simulink model "G431_ADC"  (R2018b)
settings: Solver=FixedStepDiscrete  StartTime=0.0  StopTime=10.0  FixedStep=0.010  RelTol=1e-3  EnableMultiTasking=on
libraries: ADC_Lib x2, USART_Lib x2, STM32_Config_Lib x1
settings Model: Creator=reynaudp  LastModifiedBy=fenard1
settings DataIOCC: LimitDataPoints=on  SaveFormat=Array
settings OptimizationCC: DefaultParameterBehavior=Inlined  DefaultUnderspecifiedDataType=single  LifeSpan=1
settings DebuggingCC: UnderspecifiedInitializationDetection=Classic  MergeDetectMultiDrivingBlocksExec=none  SolverPrmCheckMsg=warning  UniqueDataStoreMsg=error  AllowSymbolicDim=off  StrictBusMsg=ErrorOnBusTreatedAsVector  SFUnexpectedBacktrackingDiag=warning  SFNoUnconditionalDefaultTransitionDiag=warning  SFUndirectedBroadcastEventsDiag=error  SFExecutionAtInitializationDiag=none
settings HardwareCC: ProdBitPerPointer=32  ProdBitPerSizeT=32  ProdBitPerPtrDiffT=32  ProdLargestAtomicInteger=Integer  ProdWordSize=32  ProdHWDeviceType=STMicroelectronics->STM32 32-bit Cortex-M  TargetBitPerPointer=64  TargetBitPerSizeT=64  TargetBitPerPtrDiffT=64  TargetLongLongMode=on  TargetIntDivRoundTo=Zero  TargetEndianess=LittleEndian  TargetWordSize=64  TargetHWDeviceType=MATLAB Host  ProdEqTarget=off
settings ModelReferenceCC: PropagateSignalLabelsOutOfModel=off
settings SFSimCC: SimUseLocalCustomCode=off  CompileTimeRecursionLimit=0  EnableRuntimeRecursion=off  MATLABDynamicMemAlloc=off
settings RTWCC: SystemTargetFile=stm32.tlc  TemplateMakefile=stm32.tmf  Description=stm32 (Embedded Target)  GenerateReport=on  RTWUseLocalCustomCode=off  IncludeHyperlinkInReport=on
settings CodeAppCC: IgnoreCustomStorageClasses=off  CustomSymbolStrType=$N$R$M  SimulinkBlockComments=off
settings STFCustomTargetCC: ParMdlRefBuildCompliant=on  IncludeMdlTerminateFcn=off  CombineOutputUpdateFcns=on  ERTCustomFileBanners=on  SupportComplex=off  SupportContinuousTime=off  SupportNonInlinedSFcns=off  RemoveResetFunc=on  ParenthesesLevel=Maximum  CastingMode=Standards  MATLABClassNameForMDSCustomization=Simulink.SoftwareTarget.ERTCustomization  SystemTargetFile=stm32.tlc
settings ERTTargetCC: MultiwordLength=2048  CompOptLevelCompliant=off  ConcurrentExecutionCompliant=off  IncludeMdlTerminateFcn=off  SupportComplex=off  ParenthesesLevel=Maximum  CastingMode=Standards  ModelStepFunctionPrototypeControlCompliant=off  CPPClassGenCompliant=off  UseToolchainInfoCompliant=off  ERTSrcFileBannerTemplate=sourceFileTemplate.cgt  ERTHdrFileBannerTemplate=sourceFileTemplate.cgt  ERTDataSrcFileTemplate=sourceFileTemplate.cgt  ERTDataHdrFileTemplate=sourceFileTemplate.cgt  ERTCustomFileTemplate=customRoutineProcess.tlc  ConvertIfToSwitch=off  SuppressUnreachableDefaultCases=off
settings ConfigComp: CovMetricSettings=dw  CovHtmlReporting=on  CovSaveCumulativeToWorkspaceVar=on  CovSaveSingleToWorkspaceVar=on  CovExternalEMLEnable=off  CovSFcnEnable=off

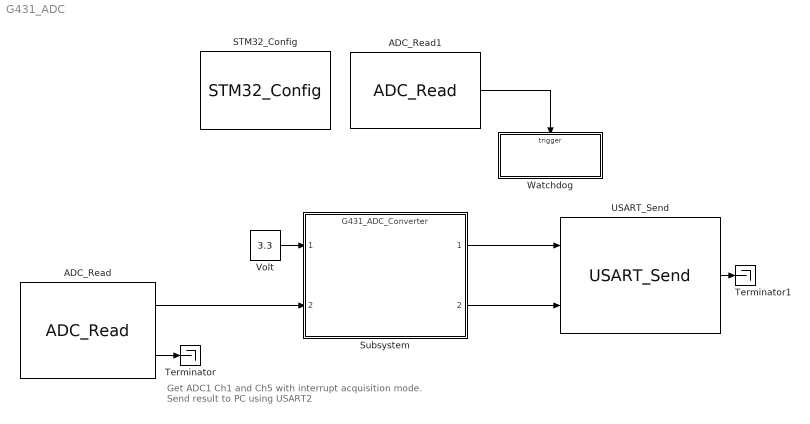
== system G431_ADC ==
  note: Get ADC1 Ch1 and Ch5 with interrupt acquisition mode.
      | Send result to PC using USART2
  ADC_Read : ADC_Lib/ADC_Read  ADC_Name=ADC1  ADC_Ch0=off  ADC_Ch1=on  ADC_Ch2=off  ADC_Ch3=off  ADC_Ch4=off  ADC_Ch5=on  ADC_Ch6=off  ADC_Ch7=off  ADC_Ch8=off  ADC_Ch9=off  ADC_Ch10=off  ADC_Ch11=off  ADC_Ch12=off  ADC_Ch13=off  ADC_Ch14=off  ADC_Ch15=off  ADC_Ch16=off  ADC_Ch17=off  ADC_Ch18=off  RgRk1=on  RgRk2=on  RgRk3=off  RgRk4=off  RgRk1_Ch=Ch1_r1  RgRk2_Ch=Ch5_r2  RgRk3_Ch=off  RgRk4_Ch=off  RgRk5=off  RgRk6=off  RgRk7=off  RgRk8=off  RgRk5_Ch=off  RgRk6_Ch=off  RgRk7_Ch=off  RgRk8_Ch=off  RgRk9=off  RgRk10=off  RgRk11=off  RgRk12=off  RgRk9_Ch=off  RgRk10_Ch=off  RgRk11_Ch=off  RgRk12_Ch=off  RgRk13=off  RgRk14=off  RgRk15=off  RgRk16=off  RgRk13_Ch=off  RgRk14_Ch=off  RgRk15_Ch=off  RgRk16_Ch=off  InjRk1=off  InjRk2=off  InjRk3=off  InjRk4=off  InjRk1_Ch=off  InjRk2_Ch=off  InjRk3_Ch=off  InjRk4_Ch=off  ADC_Trig=Not used  ADC_TrigEdge=Not used  DmaReq=off  DMA_Buffer=0  ItReq=on  AWD_Mode=SINGLE_REG  AWD_Ch=1  AWD_HThres=2000  AWD_LThres=500  AWD_En_Int=on  AWD2_HThres=0  AWD2_LThres=0  AWD2_En_Int=off  AWD3_HThres=0  AWD3_LThres=0  AWD3_En_Int=off  EOC_SEQ=off  EOC_IT=off  JEOC_IT=off  AWD_IT=off  OVR_IT=off  CpltTrans=off  HalfTrans=off  ADC_RegNb=2  ADC_RegCh0=off  ADC_RegCh1=on  ADC_RegCh2=off  ADC_RegCh3=off  ADC_RegCh4=off  ADC_RegCh5=on  ADC_RegCh6=off  ADC_RegCh7=off  ADC_RegCh8=off  ADC_RegCh9=off  ADC_RegCh10=off  ADC_RegCh11=off  ADC_RegCh12=off  ADC_RegCh13=off  ADC_RegCh14=off  ADC_RegCh15=off  ADC_RegCh16=off  ADC_RegCh17=off  ADC_RegCh18=off  ADC_InjNb=0  ADC_InjCh0=off  ADC_InjCh1=off  ADC_InjCh2=off  ADC_InjCh3=off  ADC_InjCh4=off  ADC_InjCh5=off  ADC_InjCh6=off  ADC_InjCh7=off  ADC_InjCh8=off  ADC_InjCh9=off  ADC_InjCh10=off  ADC_InjCh11=off  ADC_InjCh12=off  ADC_InjCh13=off  ADC_InjCh14=off  ADC_InjCh15=off  ADC_InjCh16=off  ADC_InjCh17=off  ADC_InjCh18=off  NbADC=1  CurrentADC=ADC1
      settings: SourceProductName=Target Support Package - STM32 Adapter
  ADC_Read1 : ADC_Lib/ADC_Read  ADC_Name=ADC1  ADC_Ch0=off  ADC_Ch1=off  ADC_Ch2=off  ADC_Ch3=off  ADC_Ch4=off  ADC_Ch5=off  ADC_Ch6=off  ADC_Ch7=off  ADC_Ch8=off  ADC_Ch9=off  ADC_Ch10=off  ADC_Ch11=off  ADC_Ch12=off  ADC_Ch13=off  ADC_Ch14=off  ADC_Ch15=off  ADC_Ch16=off  ADC_Ch17=off  ADC_Ch18=off  RgRk1=off  RgRk2=off  RgRk3=off  RgRk4=off  RgRk1_Ch=Ch1_r1  RgRk2_Ch=Ch5_r2  RgRk3_Ch=off  RgRk4_Ch=off  RgRk5=off  RgRk6=off  RgRk7=off  RgRk8=off  RgRk5_Ch=off  RgRk6_Ch=off  RgRk7_Ch=off  RgRk8_Ch=off  RgRk9=off  RgRk10=off  RgRk11=off  RgRk12=off  RgRk9_Ch=off  RgRk10_Ch=off  RgRk11_Ch=off  RgRk12_Ch=off  RgRk13=off  RgRk14=off  RgRk15=off  RgRk16=off  RgRk13_Ch=off  RgRk14_Ch=off  RgRk15_Ch=off  RgRk16_Ch=off  InjRk1=off  InjRk2=off  InjRk3=off  InjRk4=off  InjRk1_Ch=off  InjRk2_Ch=off  InjRk3_Ch=off  InjRk4_Ch=off  ADC_Trig=Not used  ADC_TrigEdge=Not used  DmaReq=off  DMA_Buffer=0  ItReq=on  AWD_Mode=SINGLE_REG  AWD_Ch=1  AWD_HThres=2000  AWD_LThres=500  AWD_En_Int=on  AWD2_HThres=0  AWD2_LThres=0  AWD2_En_Int=off  AWD3_HThres=0  AWD3_LThres=0  AWD3_En_Int=off  EOC_SEQ=off  EOC_IT=off  JEOC_IT=off  AWD_IT=on  OVR_IT=off  CpltTrans=off  HalfTrans=off  ADC_RegNb=2  ADC_RegCh0=off  ADC_RegCh1=on  ADC_RegCh2=off  ADC_RegCh3=off  ADC_RegCh4=off  ADC_RegCh5=on  ADC_RegCh6=off  ADC_RegCh7=off  ADC_RegCh8=off  ADC_RegCh9=off  ADC_RegCh10=off  ADC_RegCh11=off  ADC_RegCh12=off  ADC_RegCh13=off  ADC_RegCh14=off  ADC_RegCh15=off  ADC_RegCh16=off  ADC_RegCh17=off  ADC_RegCh18=off  ADC_InjNb=0  ADC_InjCh0=off  ADC_InjCh1=off  ADC_InjCh2=off  ADC_InjCh3=off  ADC_InjCh4=off  ADC_InjCh5=off  ADC_InjCh6=off  ADC_InjCh7=off  ADC_InjCh8=off  ADC_InjCh9=off  ADC_InjCh10=off  ADC_InjCh11=off  ADC_InjCh12=off  ADC_InjCh13=off  ADC_InjCh14=off  ADC_InjCh15=off  ADC_InjCh16=off  ADC_InjCh17=off  ADC_InjCh18=off  NbADC=1  CurrentADC=ADC1
      settings: SourceProductName=Target Support Package - STM32 Adapter
  STM32_Config : STM32_Config_Lib/STM32_Config  Priority=0  Project_Path=.\  Config_File=G431_ADC.ioc  MCU_Name=STM32G431RBTx
      settings: SourceProductName=Target Support Package - STM32 Adapter
  Subsystem : ModelReference  ModelNameDialog=G431_ADC_Converter.slx  SimulationMode=Normal  ModelReferenceVersion=1.203
  Terminator : Terminator
  Terminator1 : Terminator
  USART_Send : USART_Lib/USART_Send  USART_name=USART2  Buff_size=512  nbUsart=1  usartMode=Asynchronous  usartDma_Rx=off  usartDma_Tx=off  usartIt=off
      settings: SourceProductName=Target Support Package - STM32 Adapter
  Volt : Constant  Value=3.3  OutDataTypeStr=double
  Watchdog : Subsystem  TreatAsAtomicUnit=on
  wires:
  ADC_Read1/1 -> Watchdog/Trigger
  ADC_Read/2 -> Terminator/1
  USART_Send/1 -> Terminator1/1
  Volt/1 -> Subsystem/1
  ADC_Read/1 -> Subsystem/2
  Subsystem/1 -> USART_Send/1
  Subsystem/2 -> USART_Send/2

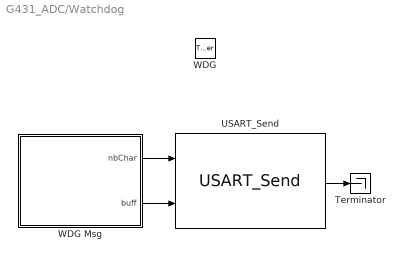
== system G431_ADC/Watchdog ==
  WDG : TriggerPort  TriggerType=function-call  VariantControl=Variant
  Terminator : Terminator
  USART_Send : USART_Lib/USART_Send  USART_name=USART2  Buff_size=128  nbUsart=1  usartMode=Asynchronous  usartDma_Rx=off  usartDma_Tx=off  usartIt=off
      settings: SourceProductName=Target Support Package - STM32 Adapter
  WDG Msg : MATLAB Function  TreatAsAtomicUnit=on
      settings: RTWSystemCode=Inline
  wires:
  WDG Msg/1(nbChar) -> USART_Send/1
  WDG Msg/2(buff) -> USART_Send/2
  USART_Send/1 -> Terminator/1

== matlab function G431_ADC/Watchdog/WDG Msg ==
  data: nbChar output uint16 size=1; buff output uint32 size=1
function [nbChar, buff] = WDG_Msg()
if coder.target('Sfun')
    % Executing in MATLAB, Buff is null
    buff = uint32(0);
    nbChar = uint16(0);
else
    coder.cinclude('getBuffPtr.h');
    % Executing in the generated code.
    y = char(['Watchdog Int',13,10,0]);
    buff = coder.ceval('getBuffPtr',coder.rref(y));
    nbChar = uint16(size(y,2));
end
end
